simulink model "test_genOpt"  (R2021b)
settings: Solver=VariableStepAuto  StartTime=0.0  StopTime=10.0  RelTol=1e-3
settings Model: Creator=enric  LastModifiedBy=enric

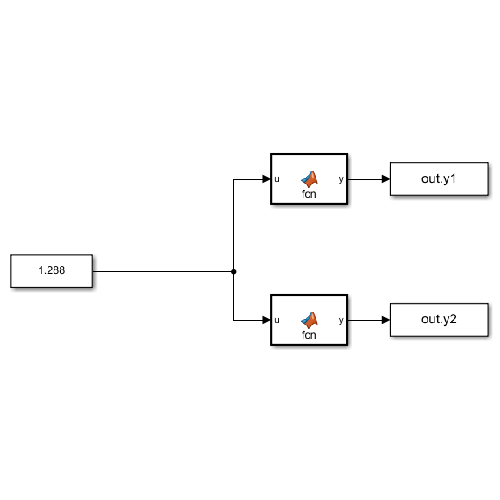
[thumbnail: Simulink's stored preview of the top-level diagram]
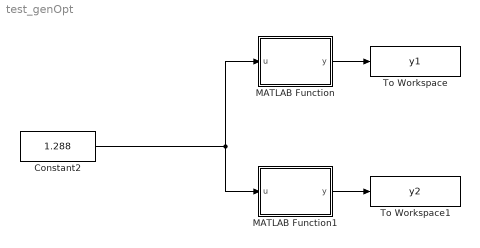
== system test_genOpt ==
  Constant2 : Constant  Value=1.288
  MATLAB Function : MATLAB Function  TreatAsAtomicUnit=on
  MATLAB Function1 : MATLAB Function  TreatAsAtomicUnit=on
  To Workspace : ToWorkspace  VariableName=y1  SampleTime=-1
  To Workspace1 : ToWorkspace  VariableName=y2  SampleTime=-1
  wires:
  Constant2/1 -> MATLAB Function1/1(u), MATLAB Function/1(u)
  MATLAB Function/1(y) -> To Workspace/1
  MATLAB Function1/1(y) -> To Workspace1/1

== matlab function test_genOpt/MATLAB Function ==
  data: u input; y output
function y = fcn(u)

y = (u+2)^2 - 10;

== matlab function test_genOpt/MATLAB Function1 ==
  data: u input; y output
function y = fcn(u)

y = (u-2)^2 + 20;
